simulink model "ThreeSines_DrSaher"  (R2018a)
settings: Solver=FixedStepDiscrete  StartTime=0.0  StopTime=0.1  RelTol=1e-3
InitFcn:
  | ST = 2e-8
  | Ts = 2e-8
libraries: simulink x10, hdlsllib x8, powerlib x1
(part 1 of 2)
settings Model: SimulationMode=accelerator  Creator=aaala  LastModifiedBy=aaala
settings OptimizationCC: BlockReduction=off  ConditionallyExecuteInputs=off  DefaultParameterBehavior=Inlined
settings DebuggingCC: AlgebraicLoopMsg=error  SingleTaskRateTransMsg=error
settings HardwareCC: ProdBitPerPointer=32  ProdBitPerSizeT=32  ProdBitPerPtrDiffT=32  ProdLargestAtomicFloat=None  ProdIntDivRoundTo=Undefined  ProdEndianess=Unspecified  ProdWordSize=32  ProdHWDeviceType=ASIC/FPGA->ASIC/FPGA  TargetBitPerPointer=64  TargetBitPerSizeT=64  TargetBitPerPtrDiffT=64  TargetLongLongMode=on  TargetIntDivRoundTo=Zero  TargetEndianess=LittleEndian  TargetWordSize=64  TargetHWDeviceType=Custom Processor->MATLAB Host Computer  ProdEqTarget=off

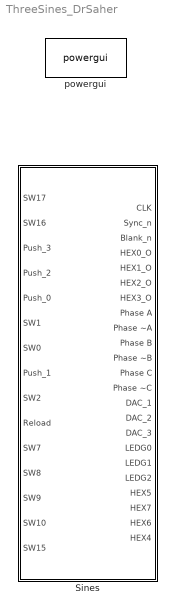
== system ThreeSines_DrSaher ==
  "Sines " : Subsystem
  powergui : powerlib/powergui  Priority=1  SimulationMode=Discrete  SampleTime=ST  frequency=60  Iterations=50  frequencyindice=60  Pbase=100e6  ErrMax=1e-4  UnitsV=kV  UnitsW=MW  buscounter=0  FunctionMessages=off  echomessages=off  EnableUseOfTLC=off  CurrentSourceSwitches=off  DisableSnubberDevices=off  DisableRonSwitches=off  DisableVfSwitches=off  DisplayEquations=off  SolverType=Tustin/Backward Euler (TBE)  Interpol=off  ExternalGateDelay=off  methode=off  Ts=100  x0status=blocks  SPID=on  SwTol=0  HookPort=off  RestoreLinks=warning  ResistiveCurrentMeasurement=off  Frange=[0:2:500]  Ylog=off  Xlog=on  ShowGrid=off  save=off  variable=ZData  structure=0  ZoomFFT=off  StartTime=0.0  cycles=1  DisplayStyle=1  fundamental=60  FreqAxis=off  MaxFrequency=1000  frequencyindicesteady=1  RmsSteady=1  display=off

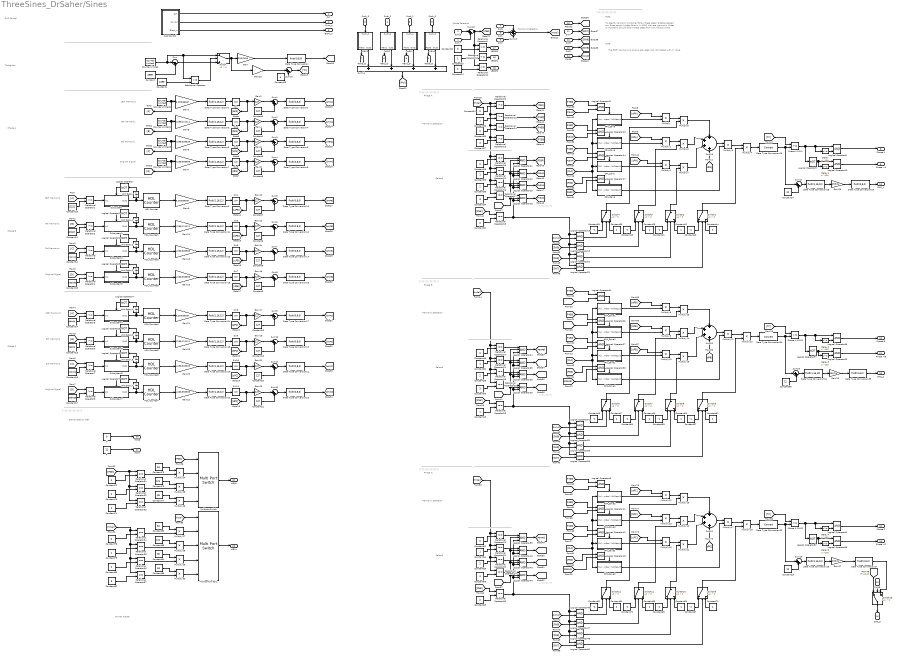
== system ThreeSines_DrSaher/Sines  ==
  note: Ahmad Alastal
  note: Phase A
  note: Phase Selection
  note: Original Signal
  note: -----------------------------------------------------------------------------------------------------------------------------------
  note: Phase A
  note: Triangular
  note: DAC Control
  note: Phase B
  note: Phase C
  note: -----------------------------------------------------------------------------------------------------------------------------------
  note: -----------------------------------------------------------------------------------------------------------------------------------
  note: -----------------------------------------------------------------------------------------------------------------------------------
  note: -----------------------------------------------------------------------------------------------------------------------------------
  note: 3rd Harmonic
  note: 9th Harmonic
  note: 15th Harmonic
  note: Original Signal
  note: 3rd Harmonic
  note: 9th Harmonic
  note: 15th Harmonic
  note: Original Signal
  note: 3rd Harmonic
  note: 9th Harmonic
  note: 15th Harmonic
  note: Harmonic Selection
  note: To specify harmonic multiplier follow these steps:
      | Disable Reload pin.
      | Enter some number [shown in HEX].
      | Activate Harmonic.
      | Order is important, should follow these steps
      | from 1-3 without jumps
  note: The 50Hz harmonic is always activated, but not loaded
      | with m value
  note: Note:
  note: |
      | |
      | |
      | |
      | |
      | |
      | |
      | |
      | |
      | |
      | |
      | |
      | |
      | |
      | |
  note: Reload
  note: -----------------------------------------------------------------
  note: Harmonic Selection
  note: /
      | /
      | /
      | /
      | /
      | /
      | /
      | /
      | /
      | /
  note: -----------------------------------------------------------------
  note: Note:
  note: |
      | |
      | |
      | |
      | |
      | |
      | |
      | |
      | |
      | |
      | |
      | |
      | |
      | |
      | |
  note: ----------------------------------------------------------------------------------------------------------------------------------------------------------------------------------------------------------------------------------------------------------------------------------------------------------------------------------------------------------------------------------
  note: Phase B
  note: Reload
  note: -----------------------------------------------------------------
  note: Harmonic Selection
  note: /
      | /
      | /
      | /
      | /
      | /
      | /
      | /
      | /
      | /
  note: |
      | |
      | |
      | |
      | |
      | |
      | |
      | |
      | |
      | |
      | |
      | |
      | |
      | |
      | |
  note: ----------------------------------------------------------------------------------------------------------------------------------------------------------------------------------------------------------------------------------------------------------------------------------------------------------------------------------------------------------------------------------
  note: Phase C
  note: Reload
  note: -----------------------------------------------------------------
  note: Harmonic Selection
  note: /
      | /
      | /
      | /
      | /
      | /
      | /
      | /
      | /
      | /
  note: |
      | |
      | |
      | |
      | |
      | |
      | |
      | |
      | |
      | |
      | |
      | |
      | |
      | |
      | |
  note: ----------------------------------------------------------------------------------------------------------------------------------------------------------------------------------------------------------------------------------------------------------------------------------------------------------------------------------------------------------------------------------
  note: Demonstration HEX
  note: |
      | |
      | |
      | |
      | |
      | |
      | |
      | |
      | |
      | |
      | |
      | |
      | |
      | |
      | |
  "SW17 " : Inport  OutDataTypeStr=boolean  SampleTime=ST
  "SW16 " : Inport  Port=2  OutDataTypeStr=boolean  SampleTime=ST
  "Push_3 " : Inport  Port=3  SampleTime=ST
  Push_2 : Inport  Port=4  SampleTime=ST
  Push_0 : Inport  Port=5  SampleTime=ST
  SW1 : Inport  Port=6  OutDataTypeStr=boolean  SampleTime=ST
  "SW0 " : Inport  Port=7  OutDataTypeStr=boolean  SampleTime=ST
  Push_1 : Inport  Port=8  SampleTime=ST
  "SW2 " : Inport  Port=9  OutDataTypeStr=boolean  SampleTime=ST
  Reload : Inport  Port=10  SampleTime=ST
  "SW7 " : Inport  Port=11  SampleTime=ST
  SW8 : Inport  Port=12  SampleTime=ST
  SW9 : Inport  Port=13  SampleTime=ST
  SW10 : Inport  Port=14  SampleTime=ST
  SW15 : Inport  Port=15  OutDataTypeStr=boolean  SampleTime=ST
  Constant : Constant  Value=4999  OutMax=[999999]  OutDataTypeStr=uint32  SampleTime=ST
  Constant{1..3,5..9,18..21} (12 alike) : Constant  Value=127  OutDataTypeStr=uint8  SampleTime=ST
  Constant10 : Constant  Value=22222  OutMax=[22222]  OutDataTypeStr=fixdt(0,16,1)  SampleTime=ST
  Constant11 : Constant  Value=37037  OutMax=[37037]  OutDataTypeStr=fixdt(0,16,0)  SampleTime=ST
  Constant12 : Constant  Value=111111  OutMax=[111111]  OutDataTypeStr=fixdt(0,17,0)  SampleTime=ST
  Constant13 : Constant  Value=333333  OutMax=[333333]  OutDataTypeStr=fixdt(0,20,1)  SampleTime=ST
  Constant14 : Constant  Value=44444  OutMax=[44444]  OutDataTypeStr=fixdt(0,16,0)  SampleTime=ST
  Constant15 : Constant  Value=74074  OutMax=[74074]  OutDataTypeStr=fixdt(0,20,3)  SampleTime=ST
  Constant16 : Constant  Value=222222  OutMax=[222222]  OutDataTypeStr=fixdt(0,20,2)  SampleTime=ST
  Constant17 : Constant  Value=666666  OutMax=[666666]  OutDataTypeStr=fixdt(0,20,0)  SampleTime=ST
  Constant22 : Constant  Value=0  OutMax=[0]  OutDataTypeStr=uint8  SampleTime=ST
  Constant23 : Constant  OutMax=[1]  OutDataTypeStr=uint8  SampleTime=ST
  Constant24 : Constant  Value=2  OutMax=[2]  OutDataTypeStr=uint8  SampleTime=ST
  Constant25 : Constant  Value=12  OutMax=[12]  OutDataTypeStr=fixdt(1,16,11)  SampleTime=ST
  Constant{26,29..30,33,35,42,44,46..47,49..50,53..54,59,61,64,69,71,73,79} (20 alike) : Constant  OutMax=[1]  OutDataTypeStr=fixdt(1,16,14)  SampleTime=ST
  Constant27 : Constant  Value=12  OutMax=[12]  OutDataTypeStr=fixdt(1,16,11)  SampleTime=ST
  Constant{28,32,34,45,52,72,78} (7 alike) : Constant  Value=0  OutMax=[0]  OutDataTypeStr=fixdt(1,16,10)  SampleTime=ST
  Constant{31,40..41,43,48,57..58,60,62,67..68,70} (12 alike) : Constant  Value=-1  OutMax=[-1]  OutDataTypeStr=fixdt(1,16,14)  SampleTime=ST
  Constant{36,38,55,63,65,74,80} (7 alike) : Constant  Value=2  OutMax=[2]  OutDataTypeStr=fixdt(1,16,13)  SampleTime=ST
  Constant{37,39,56,66,81} (5 alike) : Constant  Value=3  OutMax=[3]  OutDataTypeStr=fixdt(1,16,13)  SampleTime=ST
  Constant4 : Constant  Value=2499  OutMax=[499999]  OutDataTypeStr=uint32  SampleTime=ST
  Constant75 : Constant  Value=64  OutMax=[64]  OutDataTypeStr=fixdt(0,7,0)  SampleTime=ST
  Constant76 : Constant  Value=121  OutMax=[121]  OutDataTypeStr=fixdt(0,7,0)  SampleTime=ST
  Constant77 : Constant  Value=36  OutMax=[36]  OutDataTypeStr=fixdt(0,7,0)  SampleTime=ST
  Constant82 : Constant  Value=64  OutMax=[64]  OutDataTypeStr=fixdt(0,7,0)  SampleTime=ST
  Constant83 : Constant  Value=121  OutMax=[121]  OutDataTypeStr=fixdt(0,7,0)  SampleTime=ST
  Constant84 : Constant  Value=36  OutMax=[36]  OutDataTypeStr=fixdt(0,7,0)  SampleTime=ST
  Constant85 : Constant  Value=48  OutMax=[48]  OutDataTypeStr=fixdt(0,7,0)  SampleTime=ST
  Constant86 : Constant  Value=12  OutMax=[12]  OutDataTypeStr=fixdt(1,16,11)  SampleTime=ST
  Counter Limited : simulink/Sources/Counter Limited  uplimit=4999  tsamp=ST
  Counter Limited1 : simulink/Sources/Counter Limited  uplimit=111111  tsamp=ST
  Counter Limited2 : simulink/Sources/Counter Limited  uplimit=66667  tsamp=ST
  Counter Limited3 : simulink/Sources/Counter Limited  uplimit=333333  tsamp=ST
  Counter Limited4 : simulink/Sources/Counter Limited  uplimit=999999  tsamp=ST
  DAC Control : Subsystem
  Data Type Conversion{,2,4,6,8,10,12,14,16..17,19,21,23,27..28,35} (16 alike) : DataTypeConversion  OutMin=[0]  OutMax=[255]  OutDataTypeStr=fixdt(0,8,0)
  Data Type Conversion{1,3,5,7,9,11,13,15,18,20,22,24} (12 alike) : DataTypeConversion  OutMin=[0]  OutMax=[6.283]  OutDataTypeStr=fixdt(1,16,12)
  Data Type Conversion25 : DataTypeConversion  OutMin=[0]  OutMax=[24]  OutDataTypeStr=fixdt(1,16,10)
  Data Type Conversion26 : DataTypeConversion  OutMin=[0]  OutMax=[24]  OutDataTypeStr=fixdt(1,16,10)
  Data Type Conversion29 : DataTypeConversion
  Data Type Conversion30 : DataTypeConversion
  Data Type Conversion33 : DataTypeConversion
  Data Type Conversion34 : DataTypeConversion  OutMin=[0]  OutMax=[24]  OutDataTypeStr=fixdt(1,16,10)
  Delay{,1..5} (6 alike) : Delay  DelayLength=100  SampleTime=ST
  Gain : Gain  Gain=255/2499
  Gain1 : Gain  Gain=6.283/66667
  Gain{2,4,6,8,10,12,14,16..17,19,21,23} (12 alike) : Gain  Gain=127
  Gain11 : Gain  Gain=6.283/111111
  Gain13 : Gain  Gain=6.283/333333
  Gain15 : Gain  Gain=6.283/999999
  Gain18 : Gain  Gain=6.283/111111
  Gain20 : Gain  Gain=6.283/333333
  Gain22 : Gain  Gain=6.283/999999
  Gain24 : Gain  Gain=6.283/66667
  Gain25 : Gain  Gain=2/2500
  Gain26 : Gain  Gain=255/24
  Gain27 : Gain  Gain=255/24
  Gain29 : Gain  Gain=255/24
  Gain3 : Gain  Gain=6.283/111111
  Gain5 : Gain  Gain=6.283/333333
  Gain7 : Gain  Gain=6.283/999999
  Gain9 : Gain  Gain=6.283/66667
  H : Constant  Value=9  OutMax=[9]  OutDataTypeStr=fixdt(0,7,0)  SampleTime=ST
  HDL Counter : hdlsllib/Sources/HDL Counter  CountType=Count limited  CountInit=0  CountStep=1  CountMax=66667  CountFromType=Initial value  CountFrom=0  CountResetPort=off  CountLoadPort=off  CountEnbPort=on  CountDirPort=off  CountDataType=Unsigned  CountWordLen=24  CountFracLen=0  CountSampTime=ST
      settings: SourceProductBaseCode=HD
  HDL Counter1 : hdlsllib/Sources/HDL Counter  CountType=Count limited  CountInit=0  CountStep=1  CountMax=111111  CountFromType=Initial value  CountFrom=0  CountResetPort=off  CountLoadPort=off  CountEnbPort=on  CountDirPort=off  CountDataType=Unsigned  CountWordLen=24  CountFracLen=0  CountSampTime=ST
      settings: SourceProductBaseCode=HD
  HDL Counter2 : hdlsllib/Sources/HDL Counter  CountType=Count limited  CountInit=0  CountStep=1  CountMax=333333  CountFromType=Initial value  CountFrom=0  CountResetPort=off  CountLoadPort=off  CountEnbPort=on  CountDirPort=off  CountDataType=Unsigned  CountWordLen=24  CountFracLen=0  CountSampTime=ST
      settings: SourceProductBaseCode=HD
  HDL Counter3 : hdlsllib/Sources/HDL Counter  CountType=Count limited  CountInit=0  CountStep=1  CountMax=999999  CountFromType=Initial value  CountFrom=0  CountResetPort=off  CountLoadPort=off  CountEnbPort=on  CountDirPort=off  CountDataType=Unsigned  CountWordLen=24  CountFracLen=0  CountSampTime=ST
      settings: SourceProductBaseCode=HD
  HDL Counter4 : hdlsllib/Sources/HDL Counter  CountType=Count limited  CountInit=0  CountStep=1  CountMax=66667  CountFromType=Initial value  CountFrom=0  CountResetPort=off  CountLoadPort=off  CountEnbPort=on  CountDirPort=off  CountDataType=Unsigned  CountWordLen=24  CountFracLen=0  CountSampTime=ST
      settings: SourceProductBaseCode=HD
  HDL Counter5 : hdlsllib/Sources/HDL Counter  CountType=Count limited  CountInit=0  CountStep=1  CountMax=111111  CountFromType=Initial value  CountFrom=0  CountResetPort=off  CountLoadPort=off  CountEnbPort=on  CountDirPort=off  CountDataType=Unsigned  CountWordLen=24  CountFracLen=0  CountSampTime=ST
      settings: SourceProductBaseCode=HD
  HDL Counter6 : hdlsllib/Sources/HDL Counter  CountType=Count limited  CountInit=0  CountStep=1  CountMax=333333  CountFromType=Initial value  CountFrom=0  CountResetPort=off  CountLoadPort=off  CountEnbPort=on  CountDirPort=off  CountDataType=Unsigned  CountWordLen=24  CountFracLen=0  CountSampTime=ST
      settings: SourceProductBaseCode=HD
  HDL Counter7 : hdlsllib/Sources/HDL Counter  CountType=Count limited  CountInit=0  CountStep=1  CountMax=999999  CountFromType=Initial value  CountFrom=0  CountResetPort=off  CountLoadPort=off  CountEnbPort=on  CountDirPort=off  CountDataType=Unsigned  CountWordLen=24  CountFracLen=0  CountSampTime=ST
      settings: SourceProductBaseCode=HD
  HEX0 : Subsystem
  HEX1 : Subsystem
  HEX2 : Subsystem
  HEX3 : Subsystem
  Logical Operator{,1..7} (8 alike) : Logic  Operator=NOT  AllPortsSameDT=off  OutDataTypeStr=boolean
  Logical Operator{8,10,23,36,38,51} (6 alike) : Logic  IconShape=distinctive  AllPortsSameDT=off  OutDataTypeStr=boolean
  Logical Operator{11..12,15..16,24..25,28..29,39..40,43..44} (12 alike) : Logic  Inputs=3  AllPortsSameDT=off  OutDataTypeStr=boolean
  Logical Operator{13..14,17..22,26..27,30..35,41..42,45..50} (24 alike) : Logic  AllPortsSameDT=off  OutDataTypeStr=boolean
  Logical Operator37 : Logic  Operator=NOT  IconShape=distinctive  AllPortsSameDT=off  OutDataTypeStr=boolean
  Logical Operator52 : Logic  Operator=NOT  IconShape=distinctive  AllPortsSameDT=off  OutDataTypeStr=boolean
  Logical Operator9 : Logic  Operator=NOT  IconShape=distinctive  AllPortsSameDT=off  OutDataTypeStr=boolean
  Multiply{,1..23} (24 alike) : Product
  Multiply{24..30} (7 alike) : Product  OutDataTypeStr=fixdt(0,7,0)
  Multiport Switch : MultiPortSwitch  DataPortOrder=Zero-based contiguous  zeroidx=on
  Multiport Switch1 : MultiPortSwitch  DataPortOrder=Zero-based contiguous  Inputs=4  zeroidx=on
  P : Constant  Value=12  OutMax=[12]  OutDataTypeStr=fixdt(0,7,0)  SampleTime=ST
  Phase A PWM : RelationalOperator  OutDataTypeStr=boolean  RndMeth=Simplest
  Phase A PWM1 : RelationalOperator  OutDataTypeStr=boolean  RndMeth=Simplest
  Phase A PWM2 : RelationalOperator  OutDataTypeStr=boolean  RndMeth=Simplest
  Relational Operator : RelationalOperator  Operator=<=  OutDataTypeStr=boolean  RndMeth=Simplest
  Relational Operator{1..11,13..15,20} (15 alike) : RelationalOperator  OutDataTypeStr=boolean  RndMeth=Simplest
  Relational Operator{12,16..19,21..37} (22 alike) : RelationalOperator  Operator===  OutDataTypeStr=boolean  RndMeth=Simplest
  Sin{,1..11} (12 alike) : Trigonometry  ApproximationMethod=CORDIC
  Subsystem : Subsystem
  Subsystem1 : Subsystem
  Subsystem2 : Subsystem
  Subsystem3 : Subsystem
  Subsystem4 : Subsystem
  Subsystem5 : Subsystem
  Subsystem6 : Subsystem
  Subsystem7 : Subsystem
  Sum : Sum  Inputs=|-+
  Sum{1..13,17..18,23} (16 alike) : Sum  Inputs=|++
  Sum{14,19..20,22} (4 alike) : Sum  Inputs=++++
  Sum15 : Sum  Inputs=+++
  Sum16 : Sum  Inputs=|+-
  Switch{,1..13} (14 alike) : Switch  Criteria=u2 > Threshold
  Unit Delay{,1..7} (8 alike) : UnitDelay  SampleTime=-1
  aPA_Save : Subsystem  TreatAsAtomicUnit=on
  aPA_Save1 : Subsystem  TreatAsAtomicUnit=on
  aPA_Save2 : Subsystem  TreatAsAtomicUnit=on
  bPA_Save : Subsystem  TreatAsAtomicUnit=on
  bPA_Save1 : Subsystem  TreatAsAtomicUnit=on
  bPA_Save2 : Subsystem  TreatAsAtomicUnit=on
  cPA_Save : Subsystem  TreatAsAtomicUnit=on
  cPA_Save1 : Subsystem  TreatAsAtomicUnit=on
  cPA_Save2 : Subsystem  TreatAsAtomicUnit=on
  dPA_Save : Subsystem  TreatAsAtomicUnit=on
  dPA_Save1 : Subsystem  TreatAsAtomicUnit=on
  dPA_Save2 : Subsystem  TreatAsAtomicUnit=on
  "CLK " : Outport  OutDataTypeStr=boolean
  Sync_n : Outport  Port=2
  Blank_n : Outport  Port=3
  HEX0_O : Outport  Port=4
  HEX1_O : Outport  Port=5
  HEX2_O : Outport  Port=6
  HEX3_O : Outport  Port=7
  Phase A : Outport  Port=8
  Phase ~A : Outport  Port=9
  Phase B : Outport  Port=10
  Phase ~B : Outport  Port=11
  Phase C : Outport  Port=12
  Phase ~C : Outport  Port=13
  DAC_1 : Outport  Port=14
  DAC_2 : Outport  Port=15
  DAC_3 : Outport  Port=16
  LEDG0 : Outport  Port=17
  LEDG1 : Outport  Port=18
  LEDG2 : Outport  Port=19
  HEX5 : Outport  Port=20
  HEX7 : Outport  Port=21
  HEX6 : Outport  Port=22
  HEX4 : Outport  Port=23
  wires:
  Gain2/1 -> Sum1/1
  Sin/1 -> [aPA], Gain2/1
  Counter Limited2/1 -> [A], Gain1/1
  Gain1/1 -> Data Type Conversion1/1
  Sum1/1 -> Data Type Conversion2/1
  Data Type Conversion2/1 -> [aHPA]
  Constant2/1 -> Sum1/2
  Data Type Conversion1/1 -> Sin/1
  DAC Control/1("CLK ") -> "CLK "/1
  DAC Control/2(Sync_n) -> Sync_n/1
  DAC Control/3(Blank_n) -> Blank_n/1
  Data Type Conversion3/1 -> Sin1/1
  Constant1/1 -> Sum2/2
  Data Type Conversion4/1 -> [bHPA]
  Sum2/1 -> Data Type Conversion4/1
  Gain3/1 -> Data Type Conversion3/1
  Counter Limited1/1 -> [B], Gain3/1
  Sin1/1 -> [bPA], Gain4/1
  Gain4/1 -> Sum2/1
  Gain6/1 -> Sum3/1
  Sin2/1 -> [cPA], Gain6/1
  Counter Limited3/1 -> [C], Gain5/1
  Gain5/1 -> Data Type Conversion5/1
  Sum3/1 -> Data Type Conversion6/1
  Data Type Conversion6/1 -> [cHPA]
  Constant3/1 -> Sum3/2
  Data Type Conversion5/1 -> Sin2/1
  Constant/1 -> Sum/2
  Sum/1 -> Switch/3
  Constant4/1 -> Relational Operator/2
  Relational Operator/1 -> Switch/2
  Counter Limited/1 -> Relational Operator/1, Switch/1, Sum/1
  Data Type Conversion/1 -> [Tri_Out]
  Gain/1 -> Data Type Conversion/1
  Data Type Conversion7/1 -> Sin3/1
  Constant5/1 -> Sum4/2
  Data Type Conversion8/1 -> [dHPA]
  Sum4/1 -> Data Type Conversion8/1
  Gain7/1 -> Data Type Conversion7/1
  Counter Limited4/1 -> [D], Gain7/1
  Sin3/1 -> [dPA], Gain8/1
  Gain8/1 -> Sum4/1
  Gain16/1 -> Sum8/1
  Sin7/1 -> [dPB], Gain16/1
  Gain15/1 -> Data Type Conversion15/1
  Sum8/1 -> Data Type Conversion16/1
  Data Type Conversion16/1 -> [dHPB]
  Constant9/1 -> Sum8/2
  Data Type Conversion15/1 -> Sin7/1
  Data Type Conversion13/1 -> Sin6/1
  Constant8/1 -> Sum7/2
  Sum7/1 -> Data Type Conversion14/1
  Gain13/1 -> Data Type Conversion13/1
  Sin6/1 -> [cPB], Gain14/1
  Gain14/1 -> Sum7/1
  Gain12/1 -> Sum6/1
  Sin5/1 -> [bPB], Gain12/1
  Gain11/1 -> Data Type Conversion11/1
  Sum6/1 -> Data Type Conversion12/1
  Data Type Conversion12/1 -> [bHPB]
  Constant6/1 -> Sum6/2
  Data Type Conversion11/1 -> Sin5/1
  Gain9/1 -> Data Type Conversion9/1
  Constant7/1 -> Sum5/2
  Data Type Conversion10/1 -> [aHPB]
  Sum5/1 -> Data Type Conversion10/1
  Sin4/1 -> [aPB], Gain10/1
  Gain10/1 -> Sum5/1
  HDL Counter/1 -> Gain9/1
  Data Type Conversion9/1 -> Sin4/1
  Constant10/1 -> Relational Operator1/2
  [A] -> Relational Operator1/1
  Relational Operator1/1 -> Subsystem/1(In1)
  Subsystem/1(Out1) -> Unit Delay/1, HDL Counter/1
  Logical Operator/1 -> Subsystem/Enable
  Unit Delay/1 -> Logical Operator/1
  Unit Delay1/1 -> Logical Operator1/1
  Logical Operator1/1 -> Subsystem1/Enable
  Subsystem1/1(Out1) -> HDL Counter1/1, Unit Delay1/1
  Relational Operator2/1 -> Subsystem1/1(In1)
  [B] -> Relational Operator2/1
  Constant11/1 -> Relational Operator2/2
  HDL Counter1/1 -> Gain11/1
  HDL Counter2/1 -> Gain13/1
  Constant12/1 -> Relational Operator3/2
  [C] -> Relational Operator3/1
  Relational Operator3/1 -> Subsystem2/1(In1)
  Subsystem2/1(Out1) -> Unit Delay2/1, HDL Counter2/1
  Logical Operator2/1 -> Subsystem2/Enable
  Unit Delay2/1 -> Logical Operator2/1
  Unit Delay3/1 -> Logical Operator3/1
  Logical Operator3/1 -> Subsystem3/Enable
  Subsystem3/1(Out1) -> HDL Counter3/1, Unit Delay3/1
  Relational Operator4/1 -> Subsystem3/1(In1)
  [D] -> Relational Operator4/1
  Constant13/1 -> Relational Operator4/2
  HDL Counter3/1 -> Gain15/1
  HDL Counter7/1 -> Gain22/1
  Constant17/1 -> Relational Operator8/2
  [D] -> Relational Operator8/1
  Relational Operator8/1 -> Subsystem7/1(In1)
  Subsystem7/1(Out1) -> Unit Delay7/1, HDL Counter7/1
  Logical Operator7/1 -> Subsystem7/Enable
  Unit Delay7/1 -> Logical Operator7/1
  Unit Delay6/1 -> Logical Operator6/1
  Logical Operator6/1 -> Subsystem6/Enable
  Subsystem6/1(Out1) -> HDL Counter6/1, Unit Delay6/1
  Relational Operator7/1 -> Subsystem6/1(In1)
  [C] -> Relational Operator7/1
  Constant16/1 -> Relational Operator7/2
  HDL Counter6/1 -> Gain20/1
  HDL Counter5/1 -> Gain18/1
  Constant15/1 -> Relational Operator6/2
  [B] -> Relational Operator6/1
  Relational Operator6/1 -> Subsystem5/1(In1)
  Subsystem5/1(Out1) -> Unit Delay5/1, HDL Counter5/1
  Logical Operator5/1 -> Subsystem5/Enable
  Unit Delay5/1 -> Logical Operator5/1
  Unit Delay4/1 -> Logical Operator4/1
  Logical Operator4/1 -> Subsystem4/Enable
  Subsystem4/1(Out1) -> HDL Counter4/1, Unit Delay4/1
  Relational Operator5/1 -> Subsystem4/1(In1)
  [A] -> Relational Operator5/1
  Constant14/1 -> Relational Operator5/2
  Data Type Conversion24/1 -> Sin8/1
  HDL Counter4/1 -> Gain24/1
  Gain17/1 -> Sum9/1
  Sin8/1 -> [aPC], Gain17/1
  Sum9/1 -> Data Type Conversion17/1
  Data Type Conversion17/1 -> [aHPC]
  Constant19/1 -> Sum9/2
  Gain24/1 -> Data Type Conversion24/1
  Data Type Conversion18/1 -> Sin9/1
  Constant18/1 -> Sum10/2
  Data Type Conversion19/1 -> [bHPC]
  Sum10/1 -> Data Type Conversion19/1
  Gain18/1 -> Data Type Conversion18/1
  Sin9/1 -> [bPC], Gain19/1
  Gain19/1 -> Sum10/1
  Gain21/1 -> Sum11/1
  Sin10/1 -> [cPC], Gain21/1
  Gain20/1 -> Data Type Conversion20/1
  Sum11/1 -> Data Type Conversion21/1
  Data Type Conversion21/1 -> [cHPC]
  Constant20/1 -> Sum11/2
  Data Type Conversion20/1 -> Sin10/1
  Data Type Conversion22/1 -> Sin11/1
  Constant21/1 -> Sum12/2
  Data Type Conversion23/1 -> [dHPC]
  Sum12/1 -> Data Type Conversion23/1
  Gain22/1 -> Data Type Conversion22/1
  Sin11/1 -> [dPC], Gain23/1
  Gain23/1 -> Sum12/1
  "SW16 "/1 -> Sum13/1
  "SW17 "/1 -> Sum13/2
  "Push_3 "/1 -> HEX3/1(Push_3)
  Push_2/1 -> HEX2/1(Push_2)
  Push_1/1 -> HEX1/1(Push_1)
  Push_0/1 -> HEX0/1(Push_0)
  HEX0/1(HEX0) -> HEX0_O/1
  HEX1/1(HEX1) -> HEX1_O/1
  HEX2/1(HEX2) -> HEX2_O/1
  HEX3/1(HEX3) -> HEX3_O/1
  Sum14/1 -> [Mul]
  Sum13/1 -> [PSel], Relational Operator11/1, Relational Operator10/1, Relational Operator9/1
  Sum15/1 -> [HrSel]
  Constant26/1 -> Sum16/2
  Switch/1 -> Gain25/1, Gain/1
  Gain25/1 -> Sum16/1
  [Tri] -> Phase A PWM/1
  Delay/1 -> Logical Operator8/2
  Delay1/1 -> Logical Operator10/2
  Logical Operator9/1 -> Delay1/1, Logical Operator10/1
  Logical Operator10/1 -> Phase ~A/1
  Logical Operator8/1 -> Phase A/1
  Phase A PWM/1 -> Logical Operator9/1, Delay/1, Logical Operator8/1
  Data Type Conversion14/1 -> [cHPB]
  dPA_Save/1(MulResult) -> Multiply3/2
  "SW0 "/1 -> Sum15/1
  SW1/1 -> Sum15/2
  "SW2 "/1 -> Sum15/3
  Sum16/1 -> [Tri]
  HEX3/2(Out2) -> Sum14/1
  HEX2/2(out2) -> Sum14/2
  HEX1/2(Out2) -> Sum14/3
  HEX0/2(Out2) -> Sum14/4
  Reload/1 -> [Reload]
  "SW7 "/1 -> [SW7]
  SW8/1 -> [SW8]
  SW9/1 -> [SW9]
  SW10/1 -> [SW10]
  Data Type Conversion29/1 -> Sum17/1, Phase A PWM/2
  Data Type Conversion28/1 -> DAC_1/1
  Multiply/1 -> Multiply5/1
  Relational Operator14/1 -> [F450]
  Constant36/1 -> Relational Operator14/2
  Constant34/1 -> Relational Operator20/2
  [Mul] -> dPA_Save/1(MulNumber), aPA_Save/1(MulNumber), bPA_Save/1(MulNumber), cPA_Save/1(MulNumber)
  Relational Operator13/1 -> [F150]
  [Reload] -> Logical Operator11/2, Logical Operator12/2, Logical Operator15/2, Logical Operator16/2
  Relational Operator15/1 -> [F750]
  [cPA] -> Multiply2/1
  Relational Operator20/1 -> [F50]
  [bPA] -> Multiply1/1
  Relational Operator16/1 -> Logical Operator15/1
  Logical Operator15/1 -> [F450R]
  Relational Operator17/1 -> Logical Operator16/1
  Logical Operator11/1 -> [F50R]
  [aPA] -> Multiply/1
  Constant28/1 -> Relational Operator18/2
  Constant33/1 -> Relational Operator12/2
  Constant38/1 -> Relational Operator16/2
  Constant35/1 -> Relational Operator13/2
  [HrSel] -> Relational Operator18/1, Relational Operator12/1, Relational Operator16/1, Relational Operator17/1, Relational Operator15/1, Relational Operator14/1, Relational Operator13/1, Relational Operator20/1
  Constant39/1 -> Relational Operator17/2
  Logical Operator16/1 -> [F750R]
  Logical Operator12/1 -> [F150R]
  Multiply6/1 -> Sum19/2
  Constant31/1 -> Switch4/1
  [PSel] -> Relational Operator19/1
  Constant43/1 -> Switch3/1
  [SW9] -> Logical Operator19/2
  cPA_Save/1(MulResult) -> Multiply2/2
  [SW8] -> Logical Operator20/2
  Logical Operator22/1 -> Switch1/2
  Multiply1/1 -> Multiply6/1
  Switch4/1 -> Multiply5/2
  Constant42/1 -> Switch2/3
  Constant37/1 -> Relational Operator15/2
  [SW7] -> Logical Operator22/2
  Logical Operator21/1 -> aPA_Save/Enable
  [F150R] -> Logical Operator14/2
  [F750] -> Logical Operator21/1
  [F750R] -> Logical Operator21/2
  Constant41/1 -> Switch2/1
  Relational Operator18/1 -> Logical Operator11/1
  Multiply4/1 -> Data Type Conversion29/1
  Logical Operator14/1 -> cPA_Save/Enable
  [SW10] -> Logical Operator18/2
  [F150] -> Logical Operator14/1
  Multiply3/1 -> Multiply4/1
  Constant44/1 -> Switch1/3
  aPA_Save/1(MulResult) -> Multiply/2
  Switch2/1 -> Multiply7/2
  Sum19/1 -> Multiply3/1
  Relational Operator19/1 -> Logical Operator22/1, Logical Operator20/1, Logical Operator19/1, Logical Operator18/1, Logical Operator11/3, Logical Operator12/3, Logical Operator15/3, Logical Operator16/3
  Constant29/1 -> Switch3/3
  Switch3/1 -> Multiply6/2
  Constant30/1 -> Switch4/3
  Multiply7/1 -> Sum19/3
  Logical Operator20/1 -> Switch2/2
  Logical Operator13/1 -> bPA_Save/Enable
  Logical Operator19/1 -> Switch3/2
  Switch1/1 -> Multiply4/2
  [F50R] -> Logical Operator17/2
  Constant40/1 -> Switch1/1
  Multiply2/1 -> Multiply7/1
  [F50] -> Logical Operator17/1
  [F450] -> Logical Operator13/1
  Logical Operator18/1 -> Switch4/2
  [F450R] -> Logical Operator13/2
  Constant32/1 -> Relational Operator19/2
  bPA_Save/1(MulResult) -> Multiply1/2
  [dPA] -> Sum19/4
  Relational Operator12/1 -> Logical Operator12/1
  Multiply5/1 -> Sum19/1
  Logical Operator17/1 -> dPA_Save/Enable
  Logical Operator30/1 -> dPA_Save1/Enable
  Multiply13/1 -> Sum20/1
  Relational Operator21/1 -> Logical Operator25/1
  dPA_Save1/1(MulResult) -> Multiply11/2
  [dPB] -> Sum20/4
  bPA_Save1/1(MulResult) -> Multiply9/2
  Constant49/1 -> Relational Operator28/2
  [F450RB] -> Logical Operator26/2
  Logical Operator31/1 -> Switch8/2
  [F450] -> Logical Operator26/1
  [F50] -> Logical Operator30/1
  Multiply10/1 -> Multiply15/1
  Constant57/1 -> Switch5/1
  [F50RB] -> Logical Operator30/2
  Switch5/1 -> Multiply12/2
  Logical Operator32/1 -> Switch7/2
  Logical Operator26/1 -> bPA_Save1/Enable
  Logical Operator33/1 -> Switch6/2
  Multiply15/1 -> Sum20/3
  Constant47/1 -> Switch8/3
  Switch7/1 -> Multiply14/2
  Constant46/1 -> Switch7/3
  Relational Operator28/1 -> Logical Operator29/3, Logical Operator28/3, Logical Operator25/3, Logical Operator24/3, Logical Operator31/1, Logical Operator32/1, Logical Operator33/1, Logical Operator35/1
  Sum20/1 -> Multiply11/1
  Switch6/1 -> Multiply15/2
  aPA_Save1/1(MulResult) -> Multiply8/2
  Constant61/1 -> Switch5/3
  Multiply11/1 -> Multiply12/1
  [F150] -> Logical Operator27/1
  [SW10] -> Logical Operator31/2
  Logical Operator27/1 -> cPA_Save1/Enable
  Multiply12/1 -> Data Type Conversion30/1
  Relational Operator27/1 -> Logical Operator24/1
  Constant58/1 -> Switch6/1
  [F750RB] -> Logical Operator34/2
  [F750] -> Logical Operator34/1
  [F150RB] -> Logical Operator27/2
  Logical Operator34/1 -> aPA_Save1/Enable
  [SW7] -> Logical Operator35/2
  Constant59/1 -> Switch6/3
  Switch8/1 -> Multiply13/2
  Multiply9/1 -> Multiply14/1
  Logical Operator35/1 -> Switch5/2
  [SW8] -> Logical Operator33/2
  cPA_Save1/1(MulResult) -> Multiply10/2
  [SW9] -> Logical Operator32/2
  Constant60/1 -> Switch7/1
  [PSel] -> Relational Operator28/1
  Constant48/1 -> Switch8/1
  Multiply14/1 -> Sum20/2
  Logical Operator25/1 -> [F150RB]
  Logical Operator29/1 -> [F750RB]
  Constant56/1 -> Relational Operator26/2
  [HrSel] -> Relational Operator26/1, Relational Operator25/1, Relational Operator21/1, Relational Operator27/1
  Constant55/1 -> Relational Operator25/2
  Constant50/1 -> Relational Operator21/2
  Constant45/1 -> Relational Operator27/2
  [aPB] -> Multiply8/1
  Logical Operator24/1 -> [F50RB]
  Relational Operator26/1 -> Logical Operator29/1
  Logical Operator28/1 -> [F450RB]
  Relational Operator25/1 -> Logical Operator28/1
  [bPB] -> Multiply9/1
  [cPB] -> Multiply10/1
  [Reload] -> Logical Operator29/2, Logical Operator28/2, Logical Operator25/2, Logical Operator24/2
  [Mul] -> dPA_Save1/1(MulNumber), cPA_Save1/1(MulNumber), bPA_Save1/1(MulNumber), aPA_Save1/1(MulNumber)
  Multiply8/1 -> Multiply13/1
  Data Type Conversion35/1 -> DAC_2/1
  Phase A PWM1/1 -> Logical Operator36/1, Delay2/1, Logical Operator37/1
  Logical Operator37/1 -> Logical Operator23/1, Delay3/1
  Delay3/1 -> Logical Operator23/2
  Delay2/1 -> Logical Operator36/2
  [Tri] -> Phase A PWM1/1
  Logical Operator36/1 -> Phase B/1
  Logical Operator23/1 -> Phase ~B/1
  Logical Operator38/1 -> Phase ~C/1
  Logical Operator51/1 -> Phase C/1
  [Tri] -> Phase A PWM2/1
  Delay4/1 -> Logical Operator51/2
  Delay5/1 -> Logical Operator38/2
  Logical Operator52/1 -> Delay5/1, Logical Operator38/1
  Phase A PWM2/1 -> Logical Operator52/1, Delay4/1, Logical Operator51/1
  Multiply22/1 -> Multiply19/1
  [Mul] -> aPA_Save2/1(MulNumber), bPA_Save2/1(MulNumber), cPA_Save2/1(MulNumber), dPA_Save2/1(MulNumber)
  [Reload] -> Logical Operator39/2, Logical Operator40/2, Logical Operator43/2, Logical Operator44/2
  [cPC] -> Multiply16/1
  [bPC] -> Multiply23/1
  Relational Operator23/1 -> Logical Operator43/1
  Logical Operator43/1 -> [F450RC]
  Relational Operator24/1 -> Logical Operator44/1
  Logical Operator39/1 -> [F50RC]
  [aPC] -> Multiply22/1
  Constant52/1 -> Relational Operator29/2
  Constant64/1 -> Relational Operator22/2
  Constant65/1 -> Relational Operator23/2
  [HrSel] -> Relational Operator29/1, Relational Operator22/1, Relational Operator23/1, Relational Operator24/1
  Constant66/1 -> Relational Operator24/2
  Logical Operator44/1 -> [F750RC]
  Logical Operator40/1 -> [F150RC]
  Multiply20/1 -> Sum22/2
  Constant62/1 -> Switch12/1
  [PSel] -> Relational Operator30/1
  Constant70/1 -> Switch11/1
  [SW9] -> Logical Operator47/2
  cPA_Save2/1(MulResult) -> Multiply16/2
  [SW8] -> Logical Operator48/2
  Logical Operator50/1 -> Switch9/2
  Multiply23/1 -> Multiply20/1
  Switch12/1 -> Multiply19/2
  Constant69/1 -> Switch10/3
  [SW7] -> Logical Operator50/2
  Logical Operator49/1 -> aPA_Save2/Enable
  [F150RC] -> Logical Operator42/2
  [F750] -> Logical Operator49/1
  [F750RC] -> Logical Operator49/2
  Constant68/1 -> Switch10/1
  Relational Operator29/1 -> Logical Operator39/1
  Multiply18/1 -> Data Type Conversion33/1
  Logical Operator42/1 -> cPA_Save2/Enable
  [SW10] -> Logical Operator46/2
  [F150] -> Logical Operator42/1
  Multiply17/1 -> Multiply18/1
  Constant71/1 -> Switch9/3
  aPA_Save2/1(MulResult) -> Multiply22/2
  Switch10/1 -> Multiply21/2
  Sum22/1 -> Multiply17/1
  Relational Operator30/1 -> Logical Operator50/1, Logical Operator48/1, Logical Operator47/1, Logical Operator46/1, Logical Operator39/3, Logical Operator40/3, Logical Operator43/3, Logical Operator44/3
  Constant53/1 -> Switch11/3
  Switch11/1 -> Multiply20/2
  Constant54/1 -> Switch12/3
  Multiply21/1 -> Sum22/3
  Logical Operator48/1 -> Switch10/2
  Logical Operator41/1 -> bPA_Save2/Enable
  Logical Operator47/1 -> Switch11/2
  Switch9/1 -> Multiply18/2
  [F50RC] -> Logical Operator45/2
  Constant67/1 -> Switch9/1
  Multiply16/1 -> Multiply21/1
  [F50] -> Logical Operator45/1
  [F450] -> Logical Operator41/1
  Logical Operator46/1 -> Switch12/2
  [F450RC] -> Logical Operator41/2
  Constant63/1 -> Relational Operator30/2
  bPA_Save2/1(MulResult) -> Multiply23/2
  [dPC] -> Sum22/4
  dPA_Save2/1(MulResult) -> Multiply17/2
  Relational Operator22/1 -> Logical Operator40/1
  Multiply19/1 -> Sum22/1
  Logical Operator45/1 -> dPA_Save2/Enable
  Switch13/1 -> DAC_3/1
  SW15/1 -> Switch13/2
  [Tri_Out] -> Switch13/1
  Data Type Conversion27/1 -> Switch13/3
  Constant22/1 -> Relational Operator9/2
  Constant23/1 -> Relational Operator10/2
  Constant24/1 -> Relational Operator11/2
  Relational Operator9/1 -> LEDG0/1
  Relational Operator10/1 -> LEDG1/1
  Relational Operator11/1 -> LEDG2/1
  H/1 -> HEX5/1
  P/1 -> HEX7/1
  Constant72/1 -> Relational Operator31/2
  [PSel] -> Relational Operator33/1, Relational Operator32/1, Relational Operator31/1
  Constant73/1 -> Relational Operator32/2
  Constant74/1 -> Relational Operator33/2
  Constant75/1 -> Multiply24/1
  Relational Operator31/1 -> Multiply24/2
  Constant76/1 -> Multiply25/1
  Relational Operator32/1 -> Multiply25/2
  Constant77/1 -> Multiply26/1
  Relational Operator33/1 -> Multiply26/2
  [PSel] -> Multiport Switch/1
  Multiply24/1 -> Multiport Switch/2
  Multiply26/1 -> Multiport Switch/4
  Multiply25/1 -> Multiport Switch/3
  Multiport Switch/1 -> HEX6/1
  Constant81/1 -> Relational Operator37/2
  Constant80/1 -> Relational Operator36/2
  Constant79/1 -> Relational Operator35/2
  Constant78/1 -> Relational Operator34/2
  [HrSel] -> Relational Operator37/1, Relational Operator36/1, Relational Operator35/1, Relational Operator34/1
  Relational Operator36/1 -> Multiply29/2
  Constant84/1 -> Multiply29/1
  Relational Operator35/1 -> Multiply28/2
  Constant83/1 -> Multiply28/1
  Relational Operator34/1 -> Multiply27/2
  Constant82/1 -> Multiply27/1
  Relational Operator37/1 -> Multiply30/2
  Constant85/1 -> Multiply30/1
  Multiply30/1 -> Multiport Switch1/5
  Multiply29/1 -> Multiport Switch1/4
  Multiply28/1 -> Multiport Switch1/3
  Multiply27/1 -> Multiport Switch1/2
  [HrSel] -> Multiport Switch1/1
  Multiport Switch1/1 -> HEX4/1
  Sum17/1 -> Data Type Conversion25/1
  Data Type Conversion25/1 -> Gain26/1
  Gain26/1 -> Data Type Conversion28/1
  Constant27/1 -> Sum17/2
  Data Type Conversion30/1 -> Sum23/1, Phase A PWM1/2
  Constant86/1 -> Sum23/2
  Sum23/1 -> Data Type Conversion34/1
  Gain29/1 -> Data Type Conversion35/1
  Data Type Conversion34/1 -> Gain29/1
  Data Type Conversion33/1 -> Sum18/1, Phase A PWM2/2
  Constant25/1 -> Sum18/2
  Sum18/1 -> Data Type Conversion26/1
  Gain27/1 -> Data Type Conversion27/1
  Data Type Conversion26/1 -> Gain27/1

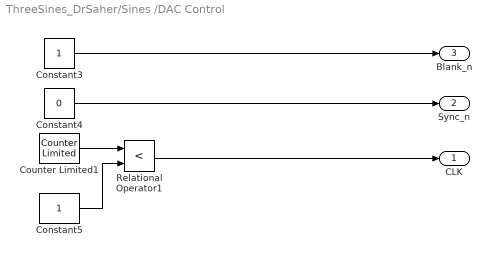
== system ThreeSines_DrSaher/Sines /DAC Control ==
  Constant3 : Constant  OutDataTypeStr=boolean  SampleTime=ST
  Constant4 : Constant  Value=0  OutDataTypeStr=boolean  SampleTime=ST
  Constant5 : Constant  OutMax=[1]  OutDataTypeStr=uint32  SampleTime=ST
  Counter Limited1 : simulink/Sources/Counter Limited  uplimit=1  tsamp=ST
  Relational Operator1 : RelationalOperator  Operator=<  OutDataTypeStr=boolean  RndMeth=Simplest
  "CLK " : Outport  OutDataTypeStr=boolean
  Sync_n : Outport  Port=2
  Blank_n : Outport  Port=3
  wires:
  Constant4/1 -> Sync_n/1
  Constant3/1 -> Blank_n/1
  Counter Limited1/1 -> Relational Operator1/1
  Relational Operator1/1 -> "CLK "/1
  Constant5/1 -> Relational Operator1/2

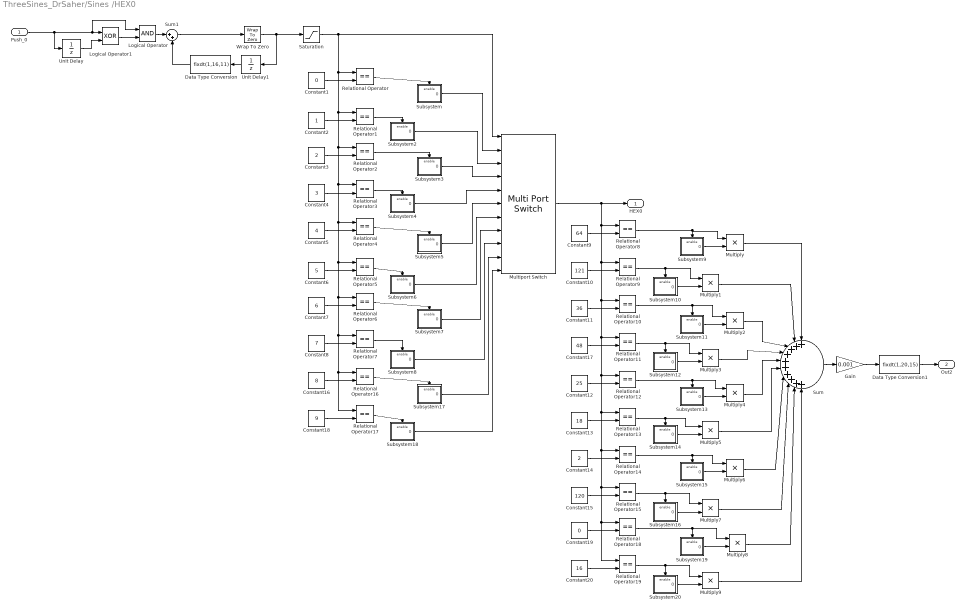
== system ThreeSines_DrSaher/Sines /HEX0 ==
  Push_0 : Inport
  Constant1 : Constant  Value=0  OutMax=[1]  OutDataTypeStr=fixdt(1,16,14)  SampleTime=Ts
  Constant10 : Constant  Value=121  OutMax=[121]  OutDataTypeStr=fixdt(0,7,0)  SampleTime=Ts
  Constant11 : Constant  Value=36  OutMax=[36]  OutDataTypeStr=fixdt(0,7,0)  SampleTime=Ts
  Constant12 : Constant  Value=25  OutMax=[25]  OutDataTypeStr=fixdt(0,7,0)  SampleTime=Ts
  Constant13 : Constant  Value=18  OutMax=[18]  OutDataTypeStr=fixdt(0,7,0)  SampleTime=Ts
  Constant14 : Constant  Value=2  OutMax=[2]  OutDataTypeStr=fixdt(0,7,0)  SampleTime=Ts
  Constant15 : Constant  Value=120  OutMax=[120]  OutDataTypeStr=fixdt(0,7,0)  SampleTime=Ts
  Constant16 : Constant  Value=8  OutMax=[8]  OutDataTypeStr=fixdt(1,16,11)  SampleTime=Ts
  Constant17 : Constant  Value=48  OutMax=[48]  OutDataTypeStr=fixdt(0,7,0)  SampleTime=Ts
  Constant18 : Constant  Value=9  OutMax=[9]  OutDataTypeStr=fixdt(1,16,11)  SampleTime=Ts
  Constant19 : Constant  Value=0  OutMax=[0]  OutDataTypeStr=fixdt(0,7,0)  SampleTime=Ts
  Constant2 : Constant  OutMax=[1]  OutDataTypeStr=fixdt(1,16,14)  SampleTime=Ts
  Constant20 : Constant  Value=16  OutMax=[16]  OutDataTypeStr=fixdt(0,7,0)  SampleTime=Ts
  Constant3 : Constant  Value=2  OutMax=[2]  OutDataTypeStr=fixdt(1,16,13)  SampleTime=Ts
  Constant4 : Constant  Value=3  OutMax=[3]  OutDataTypeStr=fixdt(1,16,13)  SampleTime=Ts
  Constant5 : Constant  Value=4  OutMax=[4]  OutDataTypeStr=fixdt(1,16,12)  SampleTime=Ts
  Constant6 : Constant  Value=5  OutMax=[5]  OutDataTypeStr=fixdt(1,16,12)  SampleTime=Ts
  Constant7 : Constant  Value=6  OutMax=[6]  OutDataTypeStr=fixdt(1,16,12)  SampleTime=Ts
  Constant8 : Constant  Value=7  OutMax=[7]  OutDataTypeStr=fixdt(1,16,12)  SampleTime=Ts
  Constant9 : Constant  Value=64  OutMax=[64]  OutDataTypeStr=fixdt(0,7,0)  SampleTime=Ts
  Data Type Conversion : DataTypeConversion  OutMax=[11]  OutDataTypeStr=fixdt(1,16,11)
  Data Type Conversion1 : DataTypeConversion  OutMax=[0.009]  OutDataTypeStr=fixdt(1,20,15)
  Gain : Gain  Gain=0.001
  Logical Operator : Logic  AllPortsSameDT=off  OutDataTypeStr=boolean
  Logical Operator1 : Logic  Operator=XOR  AllPortsSameDT=off  OutDataTypeStr=boolean
  Multiply{,1..9} (10 alike) : Product
  Multiport Switch : MultiPortSwitch  DataPortOrder=Zero-based contiguous  Inputs=10  zeroidx=on
  Relational Operator{,1..19} (20 alike) : RelationalOperator  Operator===  OutDataTypeStr=boolean  RndMeth=Nearest
  Saturation : Saturate  UpperLimit=9  LowerLimit=0
  Subsystem : Subsystem
  Subsystem10 : Subsystem
  Subsystem11 : Subsystem
  Subsystem12 : Subsystem
  Subsystem13 : Subsystem
  Subsystem14 : Subsystem
  Subsystem15 : Subsystem
  Subsystem16 : Subsystem
  Subsystem17 : Subsystem
  Subsystem18 : Subsystem
  Subsystem19 : Subsystem
  Subsystem2 : Subsystem
  Subsystem20 : Subsystem
  Subsystem3 : Subsystem
  Subsystem4 : Subsystem
  Subsystem5 : Subsystem
  Subsystem6 : Subsystem
  Subsystem7 : Subsystem
  Subsystem8 : Subsystem
  Subsystem9 : Subsystem
  Sum : Sum  Inputs=10
  Sum1 : Sum  Inputs=|++
  Unit Delay : UnitDelay  SampleTime=Ts
  Unit Delay1 : UnitDelay  SampleTime=Ts
  Wrap To Zero : simulink/Discontinuities/Wrap To Zero  Threshold=9
      settings: SourceProductName=Simulink  SourceProductBaseCode=SL
  HEX0 : Outport
  Out2 : Outport  Port=2  OutMax=[0.9]
  wires:
  Relational Operator10/1 -> Multiply2/1, Subsystem11/Enable
  Constant16/1 -> Relational Operator16/2
  Subsystem/1(0) -> Multiport Switch/2
  Relational Operator16/1 -> Subsystem17/Enable
  Subsystem15/1(0) -> Multiply6/2
  Subsystem19/1(0) -> Multiply8/2
  Multiply3/1 -> Sum/4
  Relational Operator18/1 -> Multiply8/1, Subsystem19/Enable
  Subsystem10/1(0) -> Multiply1/2
  Relational Operator13/1 -> Multiply5/1, Subsystem14/Enable
  Subsystem18/1(0) -> Multiport Switch/11
  Subsystem16/1(0) -> Multiply7/2
  Subsystem9/1(0) -> Multiply/2
  Subsystem12/1(0) -> Multiply3/2
  Constant11/1 -> Relational Operator10/2
  Relational Operator11/1 -> Multiply3/1, Subsystem12/Enable
  Multiply1/1 -> Sum/2
  Multiply5/1 -> Sum/6
  Multiport Switch/1 -> HEX0/1, Relational Operator8/1, Relational Operator11/1, Relational Operator19/1, Relational Operator18/1, Relational Operator15/1, Relational Operator14/1, Relational Operator13/1, Relational Operator12/1, Relational Operator10/1, Relational Operator9/1
  Multiply/1 -> Sum/1
  Constant19/1 -> Relational Operator18/2
  Subsystem7/1(0) -> Multiport Switch/8
  Constant3/1 -> Relational Operator2/2
  Relational Operator17/1 -> Subsystem18/Enable
  Subsystem4/1(0) -> Multiport Switch/5
  Multiply8/1 -> Sum/9
  Multiply2/1 -> Sum/3
  Constant12/1 -> Relational Operator12/2
  Relational Operator2/1 -> Subsystem3/Enable
  Constant5/1 -> Relational Operator4/2
  Constant2/1 -> Relational Operator1/2
  Subsystem3/1(0) -> Multiport Switch/4
  Relational Operator5/1 -> Subsystem6/Enable
  Relational Operator3/1 -> Subsystem4/Enable
  Constant1/1 -> Relational Operator/2
  Relational Operator1/1 -> Subsystem2/Enable
  Constant4/1 -> Relational Operator3/2
  Constant7/1 -> Relational Operator6/2
  Subsystem20/1(0) -> Multiply9/2
  Subsystem14/1(0) -> Multiply5/2
  Relational Operator12/1 -> Multiply4/1, Subsystem13/Enable
  Constant18/1 -> Relational Operator17/2
  Relational Operator14/1 -> Multiply6/1, Subsystem15/Enable
  Multiply6/1 -> Sum/7
  Constant15/1 -> Relational Operator15/2
  Multiply7/1 -> Sum/8
  Constant6/1 -> Relational Operator5/2
  Relational Operator8/1 -> Multiply/1, Subsystem9/Enable
  Relational Operator9/1 -> Multiply1/1, Subsystem10/Enable
  Subsystem8/1(0) -> Multiport Switch/9
  Subsystem5/1(0) -> Multiport Switch/6
  Constant13/1 -> Relational Operator13/2
  Constant10/1 -> Relational Operator9/2
  Multiply9/1 -> Sum/10
  Constant8/1 -> Relational Operator7/2
  Constant20/1 -> Relational Operator19/2
  Subsystem11/1(0) -> Multiply2/2
  Constant17/1 -> Relational Operator11/2
  Multiply4/1 -> Sum/5
  Relational Operator15/1 -> Subsystem16/Enable, Multiply7/1
  Subsystem2/1(0) -> Multiport Switch/3
  Relational Operator/1 -> Subsystem/Enable
  Relational Operator4/1 -> Subsystem5/Enable
  Relational Operator7/1 -> Subsystem8/Enable
  Constant14/1 -> Relational Operator14/2
  Subsystem6/1(0) -> Multiport Switch/7
  Constant9/1 -> Relational Operator8/2
  Relational Operator6/1 -> Subsystem7/Enable
  Subsystem13/1(0) -> Multiply4/2
  Relational Operator19/1 -> Subsystem20/Enable, Multiply9/1
  Subsystem17/1(0) -> Multiport Switch/10
  Saturation/1 -> Relational Operator/1, Relational Operator1/1, Relational Operator2/1, Relational Operator3/1, Relational Operator4/1, Relational Operator5/1, Relational Operator6/1, Relational Operator7/1, Relational Operator16/1, Relational Operator17/1, Multiport Switch/1
  Push_0/1 -> Unit Delay/1, Logical Operator/1, Logical Operator1/1
  Unit Delay/1 -> Logical Operator1/2
  Logical Operator1/1 -> Logical Operator/2
  Logical Operator/1 -> Sum1/1
  Unit Delay1/1 -> Data Type Conversion/1
  Sum1/1 -> Wrap To Zero/1
  Wrap To Zero/1 -> Saturation/1, Unit Delay1/1
  Data Type Conversion/1 -> Sum1/2
  Sum/1 -> Gain/1
  Gain/1 -> Data Type Conversion1/1
  Data Type Conversion1/1 -> Out2/1
